simulink subsystem "blood_compartment_flow"  (R2019b)
settings: Solver=VariableStepAuto  StartTime=0.0  StopTime=10.0  RelTol=1e-3
settings Model: Creator=RH  LastModifiedBy=RH

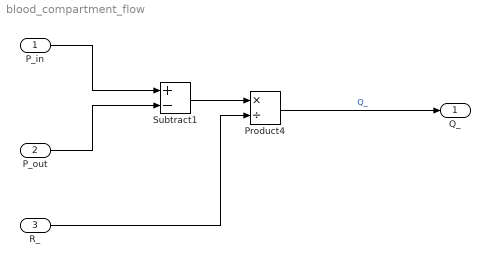
== system blood_compartment_flow ==
  P_in : Inport  Unit=mmHg
  P_out : Inport  Port=2  Unit=mmHg
  R_ : Inport  Port=3  Unit=mmHg*min/liter
  Product4 : Product  Inputs=*/
  Subtract1 : Sum  Inputs=+-
  Q_ : Outport  Unit=liter/min
  wires:
  P_in/1 -> Subtract1/1
  R_/1 -> Product4/2
  P_out/1 -> Subtract1/2
  Product4/1 -> Q_/1  "Q_"
  Subtract1/1 -> Product4/1
